simulink model "FOSTWIN"  (R2022a)
settings: Solver=FixedStepAuto  StartTime=0.0  StopTime=30  FixedStep=Ts  RelTol=1e-3
values from neighbouring files (symbols this model uses):
  D = (1+2*k*h/(sinh(2*k*h)))*tanh(k*h)    [SIDWaveGenerator.m]
  initTime = 2    [initModels_GUI.m]
  Kt = 0.943    [initModels_GUI.m]
  lpFreqCurrent = 50    [initModels_GUI.m]
  lpFreqVelocity = 50    [initModels_GUI.m]
  maxCurrent = 15    [initModels_GUI.m]
  maxFaultCount = 3    [initModels_GUI.m]
  param1 = 5    [initModels_GUI.m]    (also in starttarget.m = param1New)
  param2 = 5    [initModels_GUI.m]    (also in starttarget.m = param2New)
  param3 = 10    [initModels_GUI.m]    (also in starttarget.m = param3New)
  param4 = 10    [initModels_GUI.m]    (also in starttarget.m = param4New)
  safeDamping = 2.5    [initModels_GUI.m]
  safeTime = 20    [initModels_GUI.m]
  stableTime = 3    [initModels_GUI.m]
  Ts = 1/1000    (= 0.001)    [FOSTWINctrlPost.m]    (also in initModels_GUI.m)
  waveH = 1    [SIDWaveGenerator.m]    (also in initModels_GUI.m = 0.136; starttarget.m = waveHNew)
undefined symbols (not defined in the file or in its folder): control_id_twin4, ctrl2TwinStruct, ctrlParam1, ctrlParam2, ctrlParam3, ctrlParam4, ctrlParamStruct, curAft, curBow, dataID_twin6, param5, paramStruct, pcktID, posFlapAft, posFlapBow, SimStateMsg, state, twin2CtrlStruct
libraries: simulink x48, slrealtimeutilitieslib x24, slrealtimeethercatlib x6, slrealtimeloglib x4, dspstat3 x3, slrealtimeiplib x3, slrealtimetgmanagement x1
(part 1 of 2)
settings Model: Creator=HWRL user  LastModifiedBy=jspin
settings SolverCC: ConcurrentTasks=on  PositivePriorityOrder=on
settings DataIOCC: ExternalInput=FexAft, FexBow  TimeSaveName=toutTop  OutputSaveName=youtTop
settings OptimizationCC: BlockReduction=off  OptimizeBlockIOStorage=off  ZeroExternalMemoryAtStartup=off  ZeroInternalMemoryAtStartup=off
settings DebuggingCC: TasksWithSamePriorityMsg=none  UnconnectedInputMsg=warning  UnconnectedOutputMsg=warning  UnconnectedLineMsg=warning
settings HardwareCC: ProdBitPerLong=64  ProdLongLongMode=on  ProdHWDeviceType=Intel->x86-64 (Linux 64)
settings RTWCC: Description=Generic Real-Time Target  RTWVerbose=off  Toolchain=Simulink Real-Time Toolchain  BuildConfiguration=Faster Runs  TargetLang=C++  DLArmComputeVersion=19.05
settings GRTTargetCC: TargetLangStandard=C++03 (ISO)  CodeInterfacePackaging=C++ class

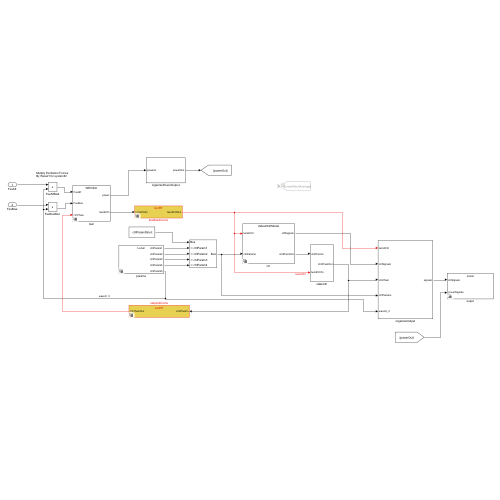
[thumbnail: Simulink's stored preview of the top-level diagram]
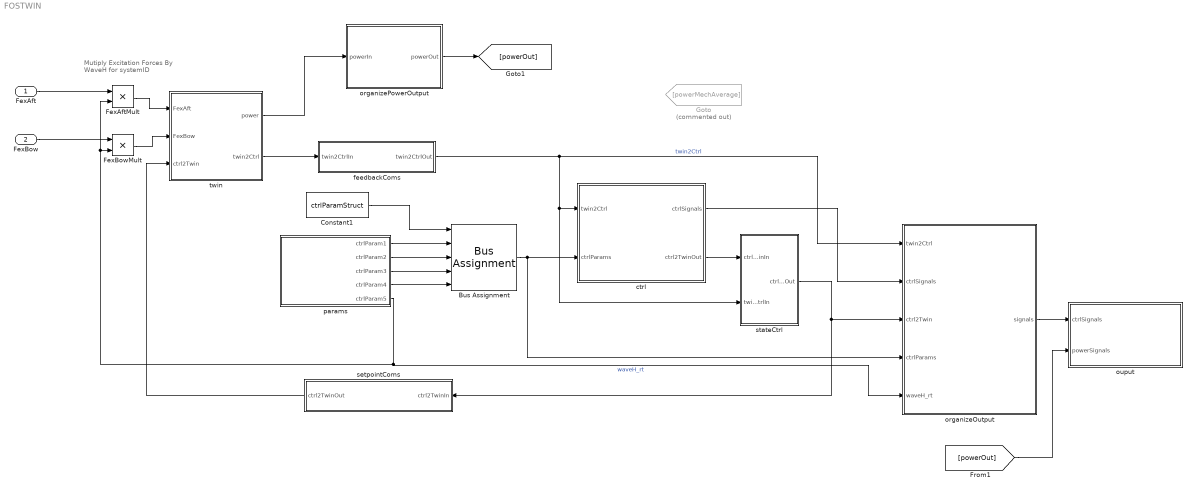
== system FOSTWIN ==
  note: Mutiply Excitation Forces
      | By WaveH for systemID
  FexAft : Inport  Interpolate=off
  FexBow : Inport  Port=2  Interpolate=off
  Bus Assignment : BusAssignment  AssignedSignals=ctrlParam1,ctrlParam2,ctrlParam3,ctrlParam4
  Constant1 : Constant  Value=ctrlParamStruct  VectorParams1D=off  OutDataTypeStr=Bus: ctrlParamBus
  FexAftMult : Product
  FexBowMult : Product
  Goto : Goto  Commented=on  GotoTag=powerMechAverage
  ctrl : Subsystem  Variant=on  VariantControlMode=label  LabelModeActiveChoice=defaultCtrlModel
  feedbackComs : Subsystem  Variant=on  VariantControlMode=label  LabelModeActiveChoice=nonRT
  organizeOutput : Subsystem
  organizePowerOutput : Subsystem
  ouput : Subsystem  Variant=on  VariantControlMode=label  LabelModeActiveChoice=Local
  params : Subsystem  Variant=on  VariantControlMode=label  LabelModeActiveChoice=Local
  setpointComs : Subsystem  Variant=on  VariantControlMode=label  LabelModeActiveChoice=nonRT
  stateCtrl : Subsystem
  twin : Subsystem  Variant=on  VariantControlMode=label  LabelModeActiveChoice=WECSim
  wires:
  FexBowMult/1 -> twin/2(FexBow)
  params/5(ctrlParam5) -> organizeOutput/5(waveH_rt), FexAftMult/2, FexBowMult/2  "waveH_rt"
  FexAftMult/1 -> twin/1(FexAft)
  setpointComs/1(ctrl2TwinOut) -> twin/3(ctrl2Twin)
  twin/2(twin2Ctrl) -> feedbackComs/1(twin2CtrlIn)
  feedbackComs/1(twin2CtrlOut) -> organizeOutput/1(twin2Ctrl), ctrl/1(twin2Ctrl), stateCtrl/2(twin2CtrlIn)  "twin2Ctrl"
  stateCtrl/1(ctrl2TwinOut) -> setpointComs/1(ctrl2TwinIn), organizeOutput/3(ctrl2Twin)
  Constant1/1 -> Bus Assignment/1
  Bus Assignment/1 -> organizeOutput/4(ctrlParams), ctrl/2(ctrlParams)
  organizeOutput/1(signals) -> ouput/1(ctrlSignals)
  twin/1(power) -> organizePowerOutput/1(powerIn)
  organizePowerOutput/1(powerOut) -> [powerOut]
  params/1(ctrlParam1) -> Bus Assignment/2
  params/2(ctrlParam2) -> Bus Assignment/3
  params/4(ctrlParam4) -> Bus Assignment/5
  [powerOut] -> ouput/2(powerSignals)
  ctrl/1(ctrlSignals) -> organizeOutput/2(ctrlSignals)
  ctrl/2(ctrl2TwinOut) -> stateCtrl/1(ctrl2TwinIn)
  params/3(ctrlParam3) -> Bus Assignment/4
  FexAft/1 -> FexAftMult/1
  FexBow/1 -> FexBowMult/1

== system FOSTWIN/ctrl ==
  note: 1) Add Subsystem or Model blocks as valid variant choices.
      | 2) You cannot connect blocks at this level. At simulation, connectivity is automatically
      | determined, based on the active variant and port name matching.
  twin2Ctrl : Inport  OutDataTypeStr=Bus: twin2CtrlBus
  ctrlParams : Inport  Port=2  OutDataTypeStr=Bus: ctrlParamBus
  defaultCtrlModel : ModelReference  ModelNameDialog=defaultCtrlModel  SimulationMode=Normal  VariantControl=defaultCtrlModel  OverrideUsingVariant=defaultCtrlModel  ModelReferenceVersion=4.551
  userCtrlModel : ModelReference  ModelNameDialog=ctrlStarter  SimulationMode=Normal  VariantControl=userCtrlModel  ModelReferenceVersion=3.17
  ctrlSignals : Outport  OutDataTypeStr=Bus: ctrlSignalBus
  ctrl2TwinOut : Outport  Port=2  OutDataTypeStr=Bus: ctrl2TwinBus

== system FOSTWIN/feedbackComs ==
  note: 1) Add Subsystem or Model blocks as valid variant choices.
      | 2) You cannot connect blocks at this level. At simulation, connectivity is automatically
      | determined, based on the active variant and port name matching.
  twin2CtrlIn : Inport  OutDataTypeStr=Bus: twin2CtrlBus
  nonRT : Subsystem  VariantControl=nonRT
  singleSpeedgoat : Subsystem  VariantControl=singleSpeedgoat
  twoSpeedgoats : Subsystem  VariantControl=twoSpeedgoats
  twin2CtrlOut : Outport  OutDataTypeStr=Bus: twin2CtrlBus

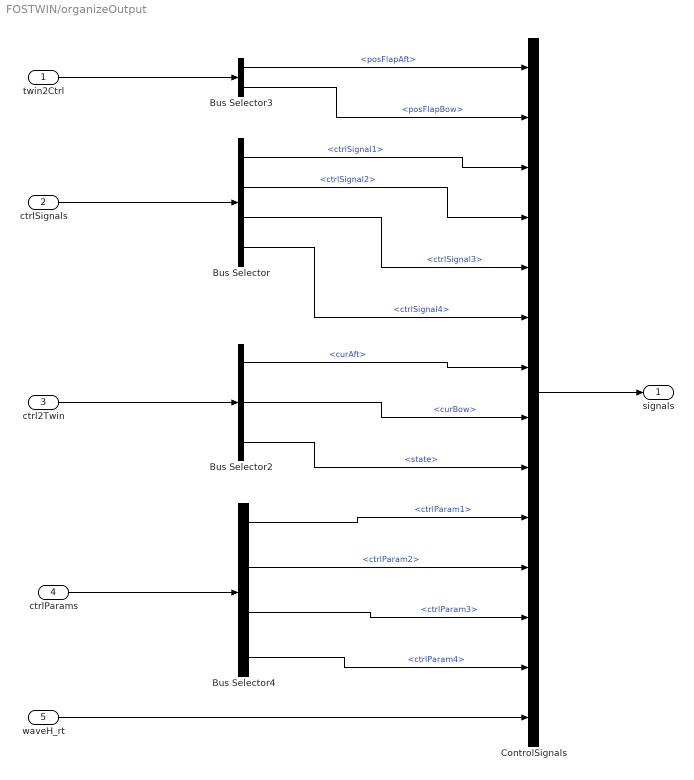
== system FOSTWIN/organizeOutput ==
  twin2Ctrl : Inport  OutDataTypeStr=Bus: twin2CtrlBus
  ctrlSignals : Inport  Port=2  OutDataTypeStr=Bus: ctrlSignalBus
  ctrl2Twin : Inport  Port=3
  ctrlParams : Inport  Port=4
  waveH_rt : Inport  Port=5
  Bus Selector : BusSelector  OutputSignals=ctrlSignal1,ctrlSignal2,ctrlSignal3,ctrlSignal4
  Bus Selector2 : BusSelector  OutputSignals=curAft,curBow,state
  Bus Selector3 : BusSelector  OutputSignals=posFlapAft,posFlapBow
  Bus Selector4 : BusSelector  OutputSignals=ctrlParam1,ctrlParam2,ctrlParam3,ctrlParam4
  ControlSignals : BusCreator  Inputs=14
  signals : Outport
  wires:
  Bus Selector2/2 -> ControlSignals/8  "<curBow>"
  waveH_rt/1 -> ControlSignals/14
  Bus Selector4/1 -> ControlSignals/10  "<ctrlParam1>"
  Bus Selector2/1 -> ControlSignals/7  "<curAft>"
  ctrlParams/1 -> Bus Selector4/1
  ControlSignals/1 -> signals/1
  ctrl2Twin/1 -> Bus Selector2/1
  twin2Ctrl/1 -> Bus Selector3/1
  Bus Selector3/1 -> ControlSignals/1  "<posFlapAft>"
  Bus Selector3/2 -> ControlSignals/2  "<posFlapBow>"
  ctrlSignals/1 -> Bus Selector/1
  Bus Selector/1 -> ControlSignals/3  "<ctrlSignal1>"
  Bus Selector/2 -> ControlSignals/4  "<ctrlSignal2>"
  Bus Selector/3 -> ControlSignals/5  "<ctrlSignal3>"
  Bus Selector/4 -> ControlSignals/6  "<ctrlSignal4>"
  Bus Selector4/2 -> ControlSignals/11  "<ctrlParam2>"
  Bus Selector4/3 -> ControlSignals/12  "<ctrlParam3>"
  Bus Selector4/4 -> ControlSignals/13  "<ctrlParam4>"
  Bus Selector2/3 -> ControlSignals/9  "<state>"

== system FOSTWIN/organizePowerOutput ==
  powerIn : Inport  OutDataTypeStr=Bus: powerBus
  Bus Creator : BusCreator  Inputs=8
  Bus Selector : BusSelector  OutputSignals=powerMechAft,powerMechBow,powerMechTotal,powerI2R,powerNet
  Bus Selector1 : BusSelector  OutputSignals=powerMechTotal
  Bus Selector2 : BusSelector  OutputSignals=powerNet
  Mean : dspstat3/Mean  run=on  InputProcessing=Columns as channels (frame based)  reset_popup=None  directionMode=Each column  dimension=1  roiEnable=off  roiType=Rectangles  roiPortion=Entire ROI  roiOutput=Individual statistics for each ROI  roiFlag=off  roundingMode=Floor  overflowMode=off  outputDataTypeStr=Inherit: Same as accumulator  outputMin=[]  outputMax=[]  outputLastDataTypeStr=Inherit: Same as accumulator
  Moving Average : dspstat3/Moving Average  Method=Sliding window  ForgettingFactorPort=off  SpecifyWindowLength=on  WindowLength=numSteps  ForgettingFactor=0.9  SimulateUsing=Code generation
  Moving Average1 : dspstat3/Moving Average  Method=Sliding window  ForgettingFactorPort=off  SpecifyWindowLength=on  WindowLength=numSteps  ForgettingFactor=0.9  SimulateUsing=Code generation
  powerOut : Outport
  wires:
  Bus Creator/1 -> powerOut/1
  Bus Selector/1 -> Bus Creator/1  "<powerMechAft>"
  Bus Selector1/1 -> Moving Average/1  "<powerMechTotal>"
  Bus Selector/3 -> Bus Creator/3  "<powerMechTotal>"
  Bus Selector/2 -> Bus Creator/2  "<powerMechBow>"
  Bus Selector/4 -> Bus Creator/4  "<powerI2R>"
  Bus Selector/5 -> Bus Creator/5  "<powerNet>"
  Moving Average/1 -> Bus Creator/6  "powerMechAverage"
  Bus Selector2/1 -> Moving Average1/1, Mean/1  "<powerNet>"
  Mean/1 -> Bus Creator/7  "powerNetMean"
  powerIn/1 -> Bus Selector2/1, Bus Selector1/1, Bus Selector/1
  Moving Average1/1 -> Bus Creator/8  "powerNetMovingAverage"

== system FOSTWIN/ouput ==
  note: 1) Add Subsystem or Model blocks as valid variant choices.
      | 2) You cannot connect blocks at this level. At simulation, connectivity is automatically
      | determined, based on the active variant and port name matching.
  ctrlSignals : Inport
  powerSignals : Inport  Port=2
  Local : Subsystem  VariantControl=Local
  Remote : Subsystem  VariantControl=Remote

== system FOSTWIN/params ==
  note: 1) Add Subsystem or Model blocks as valid variant choices.
      | 2) You cannot connect blocks at this level. At simulation, connectivity is automatically
      | determined, based on the active variant and port name matching.
  Local : Subsystem  VariantControl=Local
  Remote : Subsystem  VariantControl=Remote
  ctrlParam1 : Outport
  ctrlParam2 : Outport  Port=2
  ctrlParam3 : Outport  Port=3
  ctrlParam4 : Outport  Port=4
  ctrlParam5 : Outport  Port=5

== system FOSTWIN/setpointComs ==
  note: 1) Add Subsystem or Model blocks as valid variant choices.
      | 2) You cannot connect blocks at this level. At simulation, connectivity is automatically
      | determined, based on the active variant and port name matching.
  ctrl2TwinIn : Inport  OutDataTypeStr=Bus: ctrl2TwinBus
  nonRT : Subsystem  VariantControl=nonRT
  singleSpeedgoat : Subsystem  VariantControl=singleSpeedgoat
  twoSpeedgoats : Subsystem  VariantControl=twoSpeedgoats
  ctrl2TwinOut : Outport  OutDataTypeStr=Bus: ctrl2TwinBus

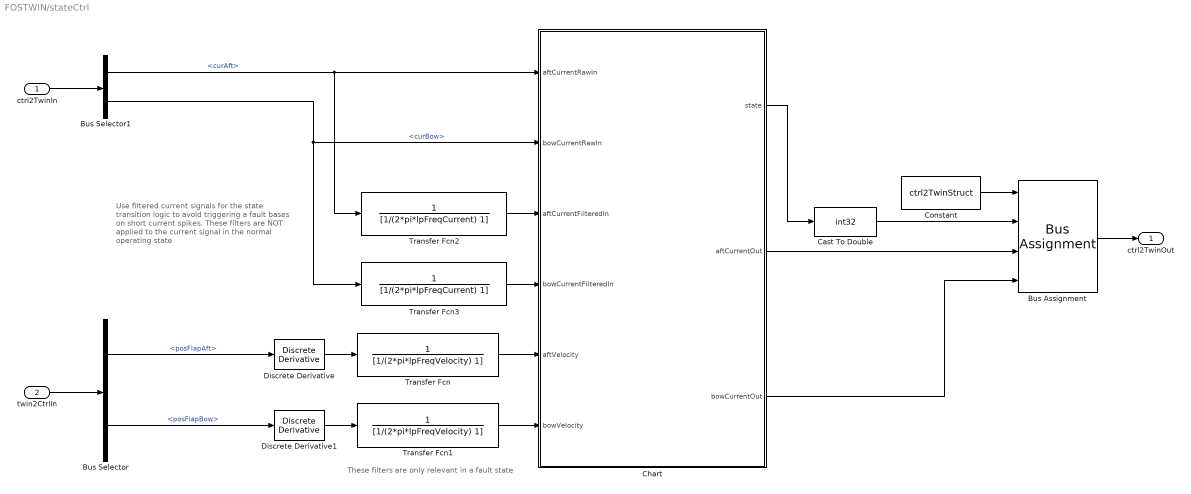
== system FOSTWIN/stateCtrl ==
  note: These filters are only relevant in a fault state
  note: Use filtered current signals for the state transition logic to avoid triggering a fault bases on short current spikes. These filters are NOT applied to the current signal in the normal operating state
  ctrl2TwinIn : Inport  OutDataTypeStr=Bus: ctrl2TwinBus
  twin2CtrlIn : Inport  Port=2  OutDataTypeStr=Bus: twin2CtrlBus
  Bus Assignment : BusAssignment  AssignedSignals=state,curAft,curBow
  Bus Selector : BusSelector  OutputSignals=posFlapAft,posFlapBow
  Bus Selector1 : BusSelector  OutputSignals=curAft,curBow
  Cast To Double : DataTypeConversion  OutDataTypeStr=int32  SaturateOnIntegerOverflow=off  RndMeth=Floor
  Chart : Stateflow chart  TreatAsAtomicUnit=on
  Constant : Constant  Value=ctrl2TwinStruct  OutDataTypeStr=Bus: ctrl2TwinBus
  Discrete Derivative : simulink/Discrete/Discrete Derivative  gainval=1.0  ICPrevScaledInput=0.0  OutMin=[]  OutMax=[]  OutDataType=fixdt(1, 16)  OutScaling=2^-10  DoSatur=off
  Discrete Derivative1 : simulink/Discrete/Discrete Derivative  gainval=1.0  ICPrevScaledInput=0.0  OutMin=[]  OutMax=[]  OutDataType=fixdt(1, 16)  OutScaling=2^-10  DoSatur=off
  Transfer Fcn : TransferFcn  Denominator=[1/(2*pi*lpFreqVelocity) 1]
  Transfer Fcn1 : TransferFcn  Denominator=[1/(2*pi*lpFreqVelocity) 1]
  Transfer Fcn2 : TransferFcn  Denominator=[1/(2*pi*lpFreqCurrent) 1]
  Transfer Fcn3 : TransferFcn  Denominator=[1/(2*pi*lpFreqCurrent) 1]
  ctrl2TwinOut : Outport  OutDataTypeStr=Bus: ctrl2TwinBus
  wires:
  Chart/1(state) -> Cast To Double/1
  Discrete Derivative/1 -> Transfer Fcn/1
  Discrete Derivative1/1 -> Transfer Fcn1/1
  Chart/3(bowCurrentOut) -> Bus Assignment/4
  Transfer Fcn/1 -> Chart/5(aftVelocity)
  Bus Selector1/1 -> Transfer Fcn2/1, Chart/1(aftCurrentRawIn)  "<curAft>"
  Transfer Fcn2/1 -> Chart/3(aftCurrentFilteredIn)
  Transfer Fcn3/1 -> Chart/4(bowCurrentFilteredIn)
  Transfer Fcn1/1 -> Chart/6(bowVelocity)
  twin2CtrlIn/1 -> Bus Selector/1
  Bus Selector/1 -> Discrete Derivative/1  "<posFlapAft>"
  Bus Selector/2 -> Discrete Derivative1/1  "<posFlapBow>"
  ctrl2TwinIn/1 -> Bus Selector1/1
  Bus Selector1/2 -> Transfer Fcn3/1, Chart/2(bowCurrentRawIn)  "<curBow>"
  Constant/1 -> Bus Assignment/1
  Chart/2(aftCurrentOut) -> Bus Assignment/3
  Bus Assignment/1 -> ctrl2TwinOut/1
  Cast To Double/1 -> Bus Assignment/2

== system FOSTWIN/twin ==
  note: 1) Add Subsystem or Model blocks as valid variant choices.
      | 2) You cannot connect blocks at this level. At simulation, connectivity is automatically
      | determined, based on the active variant and port name matching.
  FexAft : Inport
  FexBow : Inport  Port=2
  ctrl2Twin : Inport  Port=3  OutDataTypeStr=Bus: ctrl2TwinBus
  WECSim : ModelReference  ModelNameDialog=FOSWEC_v2.slx  SimulationMode=Normal  VariantControl=WECSim  ModelReferenceVersion=5.147
  systemID : ModelReference  ModelNameDialog=systemID.slx  SimulationMode=Normal  VariantControl=systemID  ModelReferenceVersion=3.515
  power : Outport  OutDataTypeStr=Bus: powerBus
  twin2Ctrl : Outport  Port=2  OutDataTypeStr=Bus: twin2CtrlBus

== system FOSTWIN/feedbackComs/nonRT ==
  twin2CtrlIn : Inport  OutDataTypeStr=Bus: twin2CtrlBus
  Memory2 : Memory
  twin2CtrlOut : Outport  OutDataTypeStr=Bus: twin2CtrlBus
  wires:
  twin2CtrlIn/1 -> Memory2/1
  Memory2/1 -> twin2CtrlOut/1

== system FOSTWIN/feedbackComs/singleSpeedgoat ==
  twin2CtrlIn : Inport  OutDataTypeStr=Bus: twin2CtrlBus
  twin2CtrlOut : Outport  OutDataTypeStr=Bus: twin2CtrlBus
  wires:
  twin2CtrlIn/1 -> twin2CtrlOut/1

== system FOSTWIN/feedbackComs/twoSpeedgoats ==
  note: TODO: Change order (aft should generally be first)
  twin2CtrlIn : Inport  OutDataTypeStr=Bus: twin2CtrlBus
  Bus Assignment : BusAssignment  AssignedSignals=posFlapBow,posFlapAft
  Constant : Constant  Value=twin2CtrlStruct  OutDataTypeStr=Bus: twin2CtrlBus
  EtherCAT Init : slrealtimeethercatlib/EtherCAT Init  Priority=0  config_file=D:\src\SANDIA-OSU\FOSTWIN-Twin\esi\FOSTWIN_Secondary1.xml  device_id=0  pci_bus=0  pci_slot=0  pci_function=0  portnum=1  initstate=2  dctuning=2  enaDebug=2  enaDC=on  errLink=off  masterDbg=off  stateChgDbg=off  baseClock=off  masterCfg=off  logFile='c:\dbglog.txt'  sample_time=0.001000  DCMode=0
      settings: SourceProductBaseCode=XP
  EtherCAT PDO Receive : slrealtimeethercatlib/EtherCAT PDO Receive  Priority=2  sig_name=Box 1 (EL6695-0002).IO Inputs.P2S01  sig_offset=328  sig_type=double  type_size=64  sig_dim=1  device_id=0  sample_time=0.001000
      settings: SourceProductBaseCode=XP
  EtherCAT PDO Receive1 : slrealtimeethercatlib/EtherCAT PDO Receive  Priority=2  sig_name=Box 1 (EL6695-0002).IO Inputs.P2S02  sig_offset=392  sig_type=double  type_size=64  sig_dim=1  device_id=0  sample_time=0.001000
      settings: SourceProductBaseCode=XP
  Terminator : Terminator
  Terminator1 : Terminator
  twin2CtrlOut : Outport
  wires:
  EtherCAT Init/1 -> Terminator/1
  twin2CtrlIn/1 -> Terminator1/1
  Constant/1 -> Bus Assignment/1
  EtherCAT PDO Receive/1 -> Bus Assignment/2
  EtherCAT PDO Receive1/1 -> Bus Assignment/3
  Bus Assignment/1 -> twin2CtrlOut/1

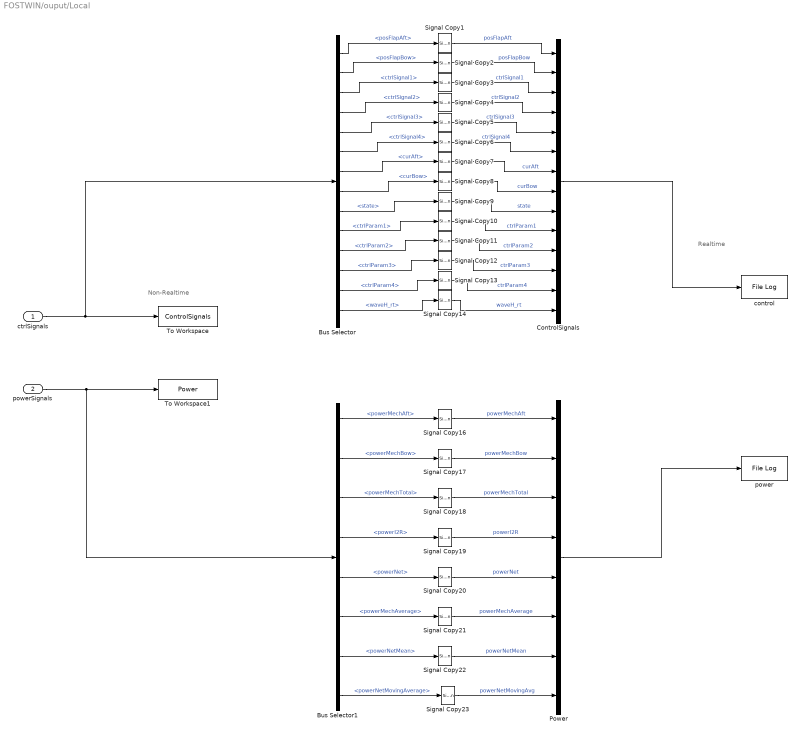
== system FOSTWIN/ouput/Local ==
  note: Non-Realtime
  note: Realtime
  ctrlSignals : Inport
  powerSignals : Inport  Port=2
  Bus Selector : BusSelector  OutputSignals=posFlapAft,posFlapBow,ctrlSignal1,ctrlSignal2,ctrlSignal3,ctrlSignal4,curAft,curBow,state,ctrlParam1,ctrlParam2,ctrlParam3,ctrlParam4,waveH_rt
  Bus Selector1 : BusSelector  OutputSignals=powerMechAft,powerMechBow,powerMechTotal,powerI2R,powerNet,powerMechAverage,powerNetMean,powerNetMovingAverage
  ControlSignals : BusCreator  Inputs=14
  Power : BusCreator  Inputs=8
  Signal Copy{1..14,16..23} (22 alike) : SignalConversion  OverrideOpt=off
  To Workspace : ToWorkspace  VariableName=ControlSignals  SaveFormat=Timeseries  SampleTime=-1
  To Workspace1 : ToWorkspace  VariableName=Power  SaveFormat=Timeseries  SampleTime=-1
  control : slrealtimeloglib/File Log  decimation=10  inputProcessing=Elements as channels (sample based)
      settings: SourceProductBaseCode=XP
  power : slrealtimeloglib/File Log  decimation=10  inputProcessing=Elements as channels (sample based)
      settings: SourceProductBaseCode=XP
  wires:
  ctrlSignals/1 -> Bus Selector/1, To Workspace/1
  powerSignals/1 -> Bus Selector1/1, To Workspace1/1
  Bus Selector/7 -> Signal Copy7/1  "<curAft>"
  Bus Selector/1 -> Signal Copy1/1  "<posFlapAft>"
  Bus Selector/2 -> Signal Copy2/1  "<posFlapBow>"
  Signal Copy1/1 -> ControlSignals/1  "posFlapAft"
  Signal Copy2/1 -> ControlSignals/2  "posFlapBow"
  Bus Selector/3 -> Signal Copy3/1  "<ctrlSignal1>"
  Bus Selector/4 -> Signal Copy4/1  "<ctrlSignal2>"
  Bus Selector/5 -> Signal Copy5/1  "<ctrlSignal3>"
  Bus Selector/6 -> Signal Copy6/1  "<ctrlSignal4>"
  Bus Selector/8 -> Signal Copy8/1  "<curBow>"
  Bus Selector/9 -> Signal Copy9/1  "<state>"
  Bus Selector/10 -> Signal Copy10/1  "<ctrlParam1>"
  Bus Selector/11 -> Signal Copy11/1  "<ctrlParam2>"
  Bus Selector/12 -> Signal Copy12/1  "<ctrlParam3>"
  Bus Selector/13 -> Signal Copy13/1  "<ctrlParam4>"
  Bus Selector/14 -> Signal Copy14/1  "<waveH_rt>"
  Signal Copy3/1 -> ControlSignals/3  "ctrlSignal1"
  Signal Copy4/1 -> ControlSignals/4  "ctrlSignal2"
  Signal Copy5/1 -> ControlSignals/5  "ctrlSignal3"
  Signal Copy6/1 -> ControlSignals/6  "ctrlSignal4"
  Signal Copy7/1 -> ControlSignals/7  "curAft"
  Signal Copy8/1 -> ControlSignals/8  "curBow"
  Signal Copy9/1 -> ControlSignals/9  "state"
  Signal Copy10/1 -> ControlSignals/10  "ctrlParam1"
  Signal Copy11/1 -> ControlSignals/11  "ctrlParam2"
  Signal Copy12/1 -> ControlSignals/12  "ctrlParam3"
  Signal Copy13/1 -> ControlSignals/13  "ctrlParam4"
  Signal Copy14/1 -> ControlSignals/14  "waveH_rt"
  ControlSignals/1 -> control/1
  Bus Selector1/6 -> Signal Copy21/1  "<powerMechAverage>"
  Bus Selector1/1 -> Signal Copy16/1  "<powerMechAft>"
  Bus Selector1/2 -> Signal Copy17/1  "<powerMechBow>"
  Bus Selector1/3 -> Signal Copy18/1  "<powerMechTotal>"
  Bus Selector1/4 -> Signal Copy19/1  "<powerI2R>"
  Bus Selector1/5 -> Signal Copy20/1  "<powerNet>"
  Signal Copy17/1 -> Power/2  "powerMechBow"
  Signal Copy18/1 -> Power/3  "powerMechTotal"
  Signal Copy19/1 -> Power/4  "powerI2R"
  Signal Copy20/1 -> Power/5  "powerNet"
  Signal Copy21/1 -> Power/6  "powerMechAverage"
  Power/1 -> power/1
  Signal Copy16/1 -> Power/1  "powerMechAft"
  Bus Selector1/7 -> Signal Copy22/1  "<powerNetMean>"
  Signal Copy22/1 -> Power/7  "powerNetMean"
  Bus Selector1/8 -> Signal Copy23/1  "<powerNetMovingAverage>"
  Signal Copy23/1 -> Power/8  "powerNetMovingAvg"

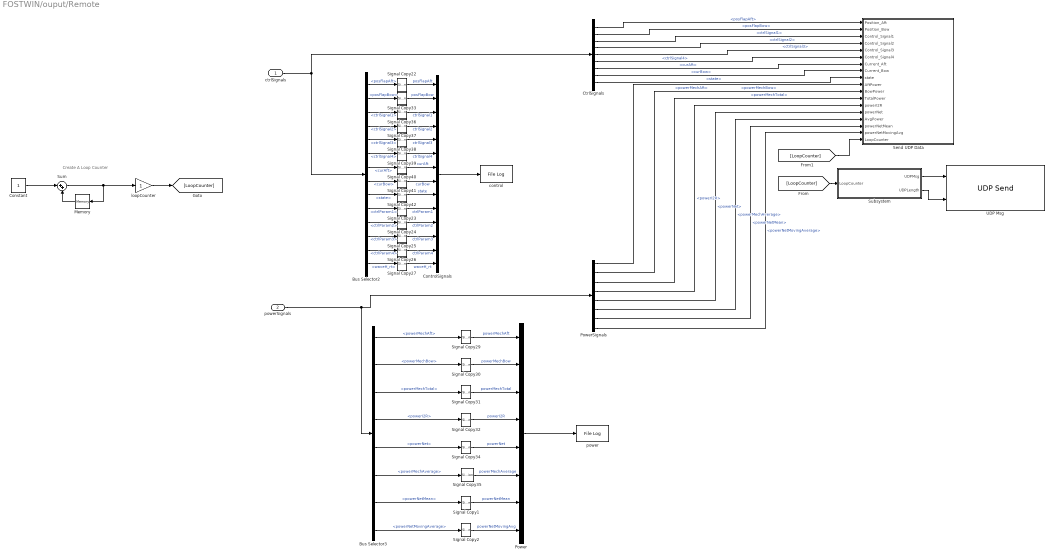
== system FOSTWIN/ouput/Remote ==
  note: Create A Loop Counter
  ctrlSignals : Inport
  powerSignals : Inport  Port=2
  Bus Selector2 : BusSelector  OutputSignals=posFlapAft,posFlapBow,ctrlSignal1,ctrlSignal2,ctrlSignal3,ctrlSignal4,curAft,curBow,state,ctrlParam1,ctrlParam2,ctrlParam3,ctrlParam4,waveH_rt
  Bus Selector3 : BusSelector  OutputSignals=powerMechAft,powerMechBow,powerMechTotal,powerI2R,powerNet,powerMechAverage,powerNetMean,powerNetMovingAverage
  Constant : Constant  SampleTime=Ts
  ControlSignals : BusCreator  Inputs=14
  CtrlSignals : BusSelector  OutputSignals=posFlapAft,posFlapBow,ctrlSignal1,ctrlSignal2,ctrlSignal3,ctrlSignal4,curAft,curBow,state
  Memory : Memory
  Power : BusCreator  Inputs=8
  PowerSignals : BusSelector  OutputSignals=powerMechAft,powerMechBow,powerMechTotal,powerI2R,powerNet,powerMechAverage,powerNetMean,powerNetMovingAverage
  Send UDP Data : Subsystem
  Signal Copy{1..2,22..27,29..42} (22 alike) : SignalConversion  OverrideOpt=off
  Subsystem : Subsystem
  Sum : Sum  Inputs=|++  OutDataTypeStr=uint32
  UDP Msg : slrealtimeiplib/UDP Send  useHostTargetConn=on  toAddress=iotIPaddr  toPort=iotRemoteMsgPort  sampleTime=Ts  enableMessage=off  ipAddress=10.10.10.15  localPort=iotLocalMsgPort
      settings: SourceProductBaseCode=XP
  control : slrealtimeloglib/File Log  decimation=10  inputProcessing=Elements as channels (sample based)
      settings: SourceProductBaseCode=XP
  loopCounter : Gain  ParamDataTypeStr=uint32  OutDataTypeStr=uint32
  power : slrealtimeloglib/File Log  decimation=10  inputProcessing=Elements as channels (sample based)
      settings: SourceProductBaseCode=XP
  wires:
  Subsystem/2(UDPLength) -> UDP Msg/2
  Sum/1 -> Memory/1, loopCounter/1
  Memory/1 -> Sum/2
  Constant/1 -> Sum/1
  Subsystem/1(UDPMsg) -> UDP Msg/1
  ctrlSignals/1 -> Bus Selector2/1, CtrlSignals/1
  CtrlSignals/1 -> Send UDP Data/1(Position_Aft)  "<posFlapAft>"
  loopCounter/1 -> [LoopCounter]
  [LoopCounter] -> Subsystem/1(LoopCounter)
  [LoopCounter] -> Send UDP Data/18(LoopCounter)
  CtrlSignals/2 -> Send UDP Data/2(Position_Bow)  "<posFlapBow>"
  CtrlSignals/3 -> Send UDP Data/3(Control_Signal1)  "<ctrlSignal1>"
  CtrlSignals/4 -> Send UDP Data/4(Control_Signal2)  "<ctrlSignal2>"
  CtrlSignals/5 -> Send UDP Data/5(Control_Signal3)  "<ctrlSignal3>"
  CtrlSignals/6 -> Send UDP Data/6(Control_Signal4)  "<ctrlSignal4>"
  CtrlSignals/7 -> Send UDP Data/7(Current_Aft)  "<curAft>"
  CtrlSignals/8 -> Send UDP Data/8(Current_Bow)  "<curBow>"
  CtrlSignals/9 -> Send UDP Data/9(state)  "<state>"
  powerSignals/1 -> PowerSignals/1, Bus Selector3/1
  PowerSignals/6 -> Send UDP Data/15(AvgPower)  "<powerMechAverage>"
  PowerSignals/5 -> Send UDP Data/14(powerNet)  "<powerNet>"
  PowerSignals/4 -> Send UDP Data/13(powerI2R)  "<powerI2R>"
  PowerSignals/3 -> Send UDP Data/12(TotalPower)  "<powerMechTotal>"
  PowerSignals/2 -> Send UDP Data/11(BowPower)  "<powerMechBow>"
  PowerSignals/1 -> Send UDP Data/10(AftPower)  "<powerMechAft>"
  Signal Copy42/1 -> ControlSignals/9  "state"
  Signal Copy31/1 -> Power/3  "powerMechTotal"
  Signal Copy32/1 -> Power/4  "powerI2R"
  Signal Copy30/1 -> Power/2  "powerMechBow"
  Signal Copy25/1 -> ControlSignals/12  "ctrlParam3"
  Signal Copy39/1 -> ControlSignals/6  "ctrlSignal4"
  Bus Selector3/5 -> Signal Copy34/1  "<powerNet>"
  Bus Selector2/5 -> Signal Copy38/1  "<ctrlSignal3>"
  Bus Selector3/2 -> Signal Copy30/1  "<powerMechBow>"
  Bus Selector2/3 -> Signal Copy36/1  "<ctrlSignal1>"
  Signal Copy36/1 -> ControlSignals/3  "ctrlSignal1"
  Signal Copy26/1 -> ControlSignals/13  "ctrlParam4"
  Bus Selector2/11 -> Signal Copy24/1  "<ctrlParam2>"
  Bus Selector3/4 -> Signal Copy32/1  "<powerI2R>"
  Signal Copy22/1 -> ControlSignals/1  "posFlapAft"
  Bus Selector2/2 -> Signal Copy33/1  "<posFlapBow>"
  Signal Copy34/1 -> Power/5  "powerNet"
  Signal Copy23/1 -> ControlSignals/10  "ctrlParam1"
  Bus Selector2/14 -> Signal Copy27/1  "<waveH_rt>"
  Signal Copy24/1 -> ControlSignals/11  "ctrlParam2"
  Bus Selector2/7 -> Signal Copy40/1  "<curAft>"
  Signal Copy41/1 -> ControlSignals/8  "curBow"
  Bus Selector3/3 -> Signal Copy31/1  "<powerMechTotal>"
  Signal Copy38/1 -> ControlSignals/5  "ctrlSignal3"
  Signal Copy37/1 -> ControlSignals/4  "ctrlSignal2"
  Signal Copy27/1 -> ControlSignals/14  "waveH_rt"
  Signal Copy40/1 -> ControlSignals/7  "curAft"
  Bus Selector2/9 -> Signal Copy42/1  "<state>"
  Bus Selector2/12 -> Signal Copy25/1  "<ctrlParam3>"
  Signal Copy35/1 -> Power/6  "powerMechAverage"
  Bus Selector2/6 -> Signal Copy39/1  "<ctrlSignal4>"
  Signal Copy29/1 -> Power/1  "powerMechAft"
  Bus Selector2/1 -> Signal Copy22/1  "<posFlapAft>"
  Bus Selector2/8 -> Signal Copy41/1  "<curBow>"
  Bus Selector2/10 -> Signal Copy23/1  "<ctrlParam1>"
  Signal Copy33/1 -> ControlSignals/2  "posFlapBow"
  Bus Selector3/1 -> Signal Copy29/1  "<powerMechAft>"
  Bus Selector2/13 -> Signal Copy26/1  "<ctrlParam4>"
  Bus Selector2/4 -> Signal Copy37/1  "<ctrlSignal2>"
  Power/1 -> power/1
  ControlSignals/1 -> control/1
  Bus Selector3/7 -> Signal Copy1/1  "<powerNetMean>"
  Signal Copy1/1 -> Power/7  "powerNetMean"
  PowerSignals/7 -> Send UDP Data/16(powerNetMean)  "<powerNetMean>"
  Bus Selector3/6 -> Signal Copy35/1  "<powerMechAverage>"
  Bus Selector3/8 -> Signal Copy2/1  "<powerNetMovingAverage>"
  Signal Copy2/1 -> Power/8  "powerNetMovingAvg"
  PowerSignals/8 -> Send UDP Data/17(powerNetMovingAvg)  "<powerNetMovingAverage>"

== system FOSTWIN/params/Local ==
  note: These Params are set in starttarget.m
  ControlParams : Subsystem  Variant=on  VariantControlMode=label  LabelModeActiveChoice=NonRealTime
  ctrlParam1 : Outport
  ctrlParam2 : Outport  Port=2
  ctrlParam3 : Outport  Port=3
  ctrlParam4 : Outport  Port=4
  ctrlParam5 : Outport  Port=5
  wires:
  ControlParams/1(ctrlParam1) -> ctrlParam1/1
  ControlParams/2(ctrlParam2) -> ctrlParam2/1
  ControlParams/3(ctrlParam3) -> ctrlParam3/1
  ControlParams/4(ctrlParam4) -> ctrlParam4/1
  ControlParams/5(ctrlParam5) -> ctrlParam5/1

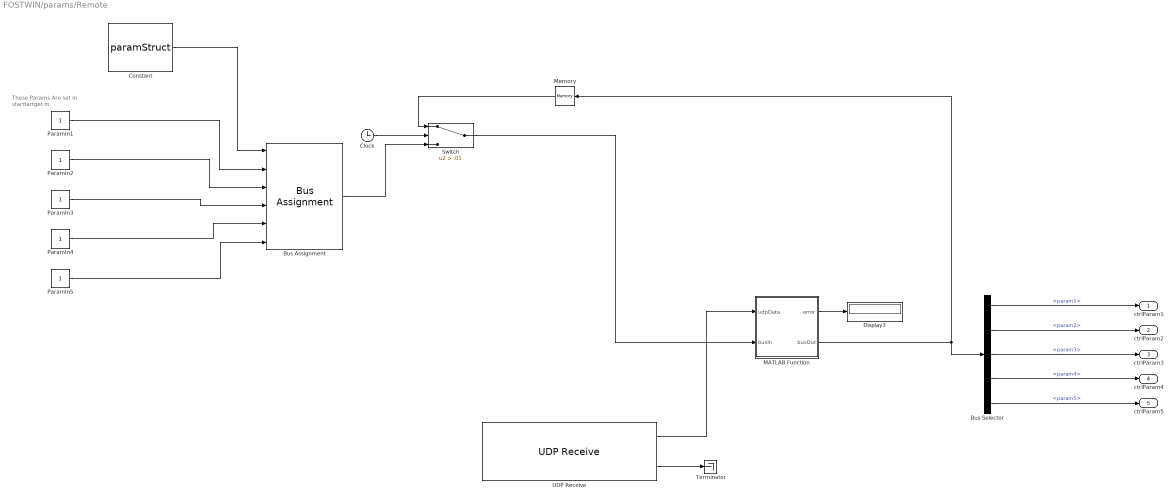
== system FOSTWIN/params/Remote ==
  note: These Params Are set in starttartget.m
  Bus Assignment : BusAssignment  AssignedSignals=param1,param2,param3,param4,param5
  Bus Selector : BusSelector  OutputSignals=param1,param2,param3,param4,param5
  Clock : Clock
  Constant : Constant  Value=paramStruct  VectorParams1D=off  OutDataTypeStr=Bus: slBus1
  Display3 : Display
  MATLAB Function : MATLAB Function  TreatAsAtomicUnit=on
  Memory : Memory
  ParamIn1 : Constant  SampleTime=Ts
  ParamIn2 : Constant  VectorParams1D=off  SampleTime=Ts
  ParamIn3 : Constant  SampleTime=Ts
  ParamIn4 : Constant  OutDataTypeStr=double  SampleTime=Ts
  ParamIn5 : Constant  OutDataTypeStr=double  SampleTime=Ts
  Switch : Switch  Criteria=u2 > Threshold  Threshold=.01  SaturateOnIntegerOverflow=off  InputSameDT=off
  Terminator : Terminator
  UDP Receive : slrealtimeiplib/UDP Receive  useHostTargetConn=on  ipAddress=10.10.10.15  localPort=iotLocalParamPort  rcvWidth=12  rcvFmAny=off  fmAddress=iotIPaddr  sampleTime=Ts  enableMessage=off  maxPackets=1
      settings: SourceProductBaseCode=XP
  ctrlParam1 : Outport
  ctrlParam2 : Outport  Port=2
  ctrlParam3 : Outport  Port=3
  ctrlParam4 : Outport  Port=4
  ctrlParam5 : Outport  Port=5
  wires:
  Bus Selector/4 -> ctrlParam4/1  "<param4>"
  Memory/1 -> Switch/1
  Bus Selector/1 -> ctrlParam1/1  "<param1>"
  UDP Receive/2 -> Terminator/1
  Bus Selector/5 -> ctrlParam5/1  "<param5>"
  UDP Receive/1 -> MATLAB Function/1(udpData)
  Clock/1 -> Switch/2
  ParamIn4/1 -> Bus Assignment/5
  MATLAB Function/1(error) -> Display3/1
  ParamIn2/1 -> Bus Assignment/3
  MATLAB Function/2(busOut) -> Memory/1, Bus Selector/1
  Switch/1 -> MATLAB Function/2(busIn)
  ParamIn3/1 -> Bus Assignment/4
  ParamIn1/1 -> Bus Assignment/2
  Bus Assignment/1 -> Switch/3
  ParamIn5/1 -> Bus Assignment/6
  Constant/1 -> Bus Assignment/1
  Bus Selector/3 -> ctrlParam3/1  "<param3>"
  Bus Selector/2 -> ctrlParam2/1  "<param2>"

== system FOSTWIN/setpointComs/nonRT ==
  ctrl2TwinIn : Inport  OutDataTypeStr=Bus: ctrl2TwinBus
  ctrl2TwinOut : Outport  OutDataTypeStr=Bus: ctrl2TwinBus
  wires:
  ctrl2TwinIn/1 -> ctrl2TwinOut/1

== system FOSTWIN/setpointComs/singleSpeedgoat ==
  ctrl2TwinIn : Inport  OutDataTypeStr=Bus: ctrl2TwinBus
  Delay2 : Delay  DelayLength=1
  ctrl2TwinOut : Outport  OutDataTypeStr=Bus: ctrl2TwinBus
  wires:
  ctrl2TwinIn/1 -> Delay2/1
  Delay2/1 -> ctrl2TwinOut/1

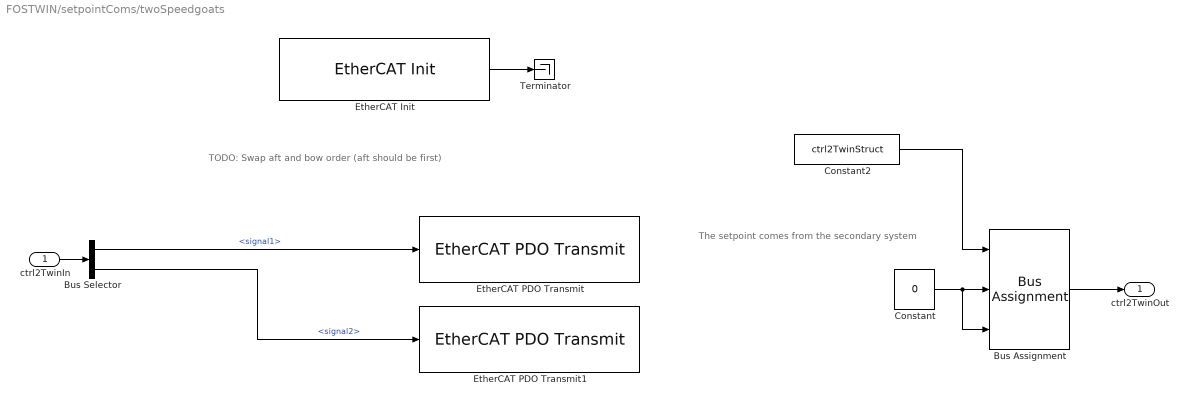
== system FOSTWIN/setpointComs/twoSpeedgoats ==
  note: TODO: Swap aft and bow order (aft should be first)
  note: The setpoint comes from the secondary system
  ctrl2TwinIn : Inport  OutDataTypeStr=Bus: ctrl2TwinBus
  Bus Assignment : BusAssignment  AssignedSignals=curAft,curBow
  Bus Selector : BusSelector  OutputSignals=signal1,signal2
  Constant : Constant  Value=0  VectorParams1D=off  SampleTime=-1
  Constant2 : Constant  Value=ctrl2TwinStruct  OutDataTypeStr=Bus: ctrl2TwinBus
  EtherCAT Init : slrealtimeethercatlib/EtherCAT Init  Priority=0  config_file=D:\src\SANDIA-OSU\FOSTWIN-Twin\esi\FOSTWIN-Primary1.xml  device_id=0  pci_bus=0  pci_slot=0  pci_function=0  portnum=1  initstate=2  dctuning=0  enaDebug=0  enaDC=on  errLink=off  masterDbg=off  stateChgDbg=off  baseClock=off  masterCfg=off  logFile='c:\dbglog.txt'  sample_time=0.001000  DCMode=0
      settings: SourceProductBaseCode=XP
  EtherCAT PDO Transmit : slrealtimeethercatlib/EtherCAT PDO Transmit  Priority=3  sig_name=Term 2 (EL6695).IO Outputs.P2S01  sig_offset=312  sig_type=double  type_size=64  sig_dim=1  device_id=0  sample_time=0.001000
      settings: SourceProductBaseCode=XP
  EtherCAT PDO Transmit1 : slrealtimeethercatlib/EtherCAT PDO Transmit  Priority=3  sig_name=Term 2 (EL6695).IO Outputs.P2S02  sig_offset=376  sig_type=double  type_size=64  sig_dim=1  device_id=0  sample_time=0.001000
      settings: SourceProductBaseCode=XP
  Terminator : Terminator
  ctrl2TwinOut : Outport
  wires:
  EtherCAT Init/1 -> Terminator/1
  Constant2/1 -> Bus Assignment/1
  Bus Assignment/1 -> ctrl2TwinOut/1
  Constant/1 -> Bus Assignment/3, Bus Assignment/2
  ctrl2TwinIn/1 -> Bus Selector/1
  Bus Selector/1 -> EtherCAT PDO Transmit/1  "<signal1>"
  Bus Selector/2 -> EtherCAT PDO Transmit1/1  "<signal2>"

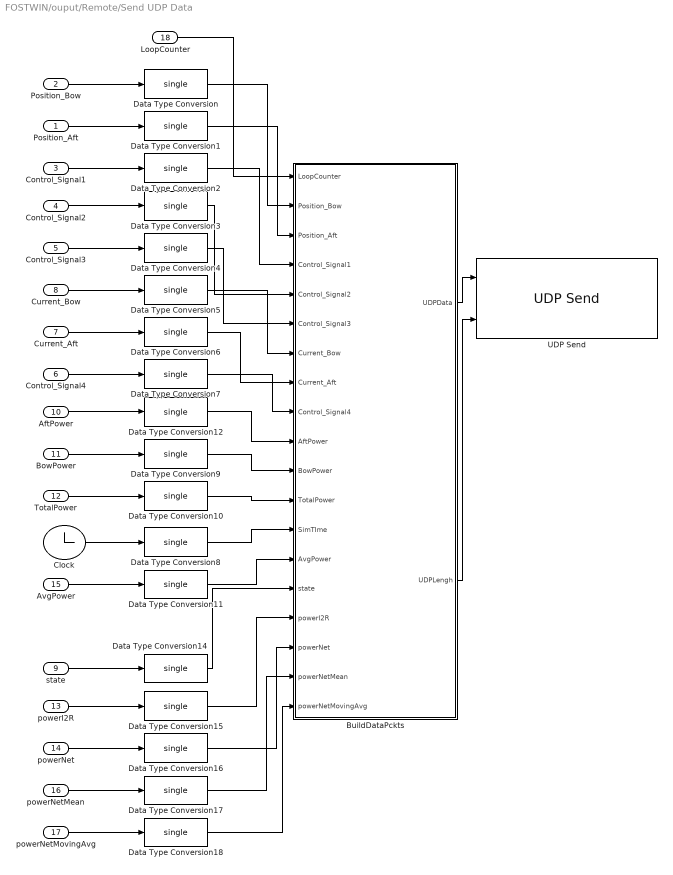
== system FOSTWIN/ouput/Remote/Send UDP Data ==
  Position_Aft : Inport
  Position_Bow : Inport  Port=2
  Control_Signal1 : Inport  Port=3
  Control_Signal2 : Inport  Port=4
  Control_Signal3 : Inport  Port=5
  Control_Signal4 : Inport  Port=6
  Current_Aft : Inport  Port=7
  Current_Bow : Inport  Port=8
  state : Inport  Port=9
  AftPower : Inport  Port=10
  BowPower : Inport  Port=11
  TotalPower : Inport  Port=12
  powerI2R : Inport  Port=13
  powerNet : Inport  Port=14
  AvgPower : Inport  Port=15
  powerNetMean : Inport  Port=16
  powerNetMovingAvg : Inport  Port=17
  LoopCounter : Inport  Port=18
  BuildDataPckts : Subsystem
  Clock : Clock
  Data Type Conversion{,1..12,14..18} (18 alike) : DataTypeConversion  OutDataTypeStr=single  SaturateOnIntegerOverflow=off  RndMeth=Floor
  UDP Send : slrealtimeiplib/UDP Send  useHostTargetConn=on  toAddress=iotIPaddr  toPort=iotRemoteDataPort  sampleTime=Ts  enableMessage=off  ipAddress=10.10.10.15  localPort=iotLocalDataPort
      settings: SourceProductBaseCode=XP
  wires:
  state/1 -> Data Type Conversion14/1
  Data Type Conversion1/1 -> BuildDataPckts/3(Position_Aft)
  Data Type Conversion16/1 -> BuildDataPckts/17(powerNet)
  Data Type Conversion15/1 -> BuildDataPckts/16(powerI2R)
  Data Type Conversion14/1 -> BuildDataPckts/15(state)
  powerI2R/1 -> Data Type Conversion15/1
  powerNet/1 -> Data Type Conversion16/1
  Data Type Conversion12/1 -> BuildDataPckts/10(AftPower)
  Data Type Conversion11/1 -> BuildDataPckts/14(AvgPower)
  Data Type Conversion10/1 -> BuildDataPckts/12(TotalPower)
  Data Type Conversion9/1 -> BuildDataPckts/11(BowPower)
  TotalPower/1 -> Data Type Conversion10/1
  AvgPower/1 -> Data Type Conversion11/1
  AftPower/1 -> Data Type Conversion12/1
  BowPower/1 -> Data Type Conversion9/1
  Data Type Conversion8/1 -> BuildDataPckts/13(SimTIme)
  Clock/1 -> Data Type Conversion8/1
  Data Type Conversion7/1 -> BuildDataPckts/9(Control_Signal4)
  Position_Aft/1 -> Data Type Conversion1/1
  LoopCounter/1 -> BuildDataPckts/1(LoopCounter)
  Current_Bow/1 -> Data Type Conversion5/1
  Control_Signal4/1 -> Data Type Conversion7/1
  Data Type Conversion5/1 -> BuildDataPckts/7(Current_Bow)
  Data Type Conversion6/1 -> BuildDataPckts/8(Current_Aft)
  Control_Signal3/1 -> Data Type Conversion4/1
  Current_Aft/1 -> Data Type Conversion6/1
  Data Type Conversion4/1 -> BuildDataPckts/6(Control_Signal3)
  Data Type Conversion3/1 -> BuildDataPckts/5(Control_Signal2)
  Control_Signal2/1 -> Data Type Conversion3/1
  Control_Signal1/1 -> Data Type Conversion2/1
  Data Type Conversion2/1 -> BuildDataPckts/4(Control_Signal1)
  Data Type Conversion/1 -> BuildDataPckts/2(Position_Bow)
  Position_Bow/1 -> Data Type Conversion/1
  BuildDataPckts/1(UDPData) -> UDP Send/1
  BuildDataPckts/2(UDPLengh) -> UDP Send/2
  powerNetMean/1 -> Data Type Conversion17/1
  Data Type Conversion17/1 -> BuildDataPckts/18(powerNetMean)
  powerNetMovingAvg/1 -> Data Type Conversion18/1
  Data Type Conversion18/1 -> BuildDataPckts/19(powerNetMovingAvg)

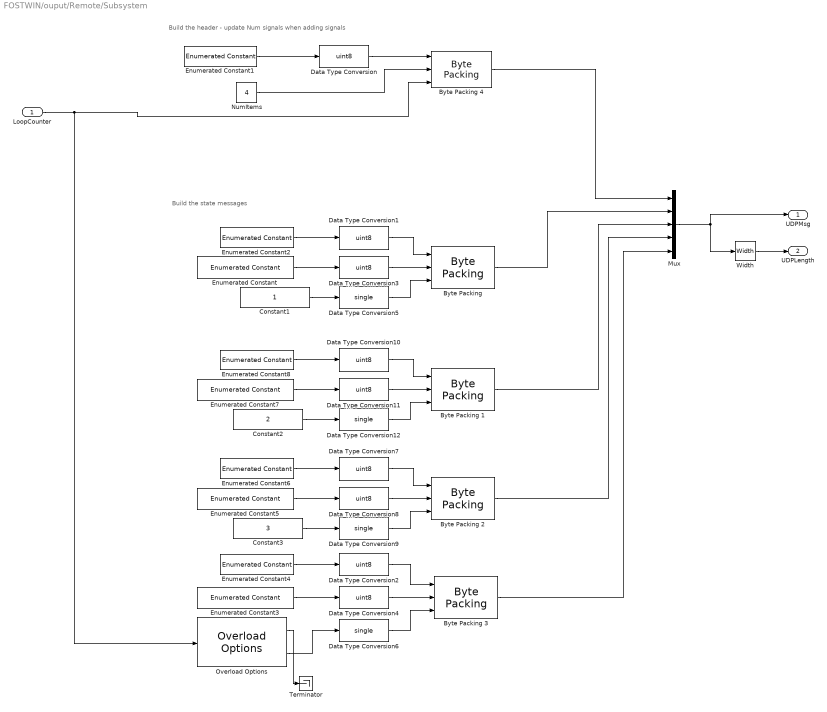
== system FOSTWIN/ouput/Remote/Subsystem ==
  note: Build the state messages
  note: Build the header - update Num signals when adding signals
  LoopCounter : Inport
  Byte Packing {,1..4} (5 alike) : slrealtimeutilitieslib/Byte Packing
  Constant1 : Constant
  Constant2 : Constant  Value=2
  Constant3 : Constant  Value=3
  Data Type Conversion{,1..4,7..8,10..11} (9 alike) : DataTypeConversion  OutDataTypeStr=uint8  SaturateOnIntegerOverflow=off  RndMeth=Floor
  Data Type Conversion{5..6,9,12} (4 alike) : DataTypeConversion  OutDataTypeStr=single  SaturateOnIntegerOverflow=off  RndMeth=Floor
  Enumerated Constant : simulink/Sources/Enumerated Constant  OutDataTypeStr=Enum: SimStateMsg  Value=SimStateMsg.eCATState  SampleTime=inf
  Enumerated Constant1 : simulink/Sources/Enumerated Constant  OutDataTypeStr=Enum: pcktID  Value=pcktID.header  SampleTime=inf
  Enumerated Constant{2,4,6,8} (4 alike) : simulink/Sources/Enumerated Constant  OutDataTypeStr=Enum: pcktID  Value=pcktID.stateMsg  SampleTime=inf
  Enumerated Constant3 : simulink/Sources/Enumerated Constant  OutDataTypeStr=Enum: SimStateMsg  Value=SimStateMsg.cpuTET  SampleTime=inf
  Enumerated Constant5 : simulink/Sources/Enumerated Constant  OutDataTypeStr=Enum: SimStateMsg  Value=SimStateMsg.eCATLastErr  SampleTime=inf
  Enumerated Constant7 : simulink/Sources/Enumerated Constant  OutDataTypeStr=Enum: SimStateMsg  Value=SimStateMsg.eCATErr  SampleTime=inf
  Mux : Mux  Inputs=5
  NumItems : Constant  Value=4  OutDataTypeStr=uint8
  Overload Options : slrealtimetgmanagement/Overload Options  startupDur=60  startupDurSrc=Tunable Parameter  maxOverload=200  maxOverloadSrc=Tunable Parameter  TETFlag=on
      settings: SourceProductBaseCode=XP
  Terminator : Terminator
  Width : Width
  UDPMsg : Outport
  UDPLength : Outport  Port=2
  wires:
  Constant2/1 -> Data Type Conversion12/1
  NumItems/1 -> Byte Packing 4/2
  Data Type Conversion9/1 -> Byte Packing 2/3
  Constant3/1 -> Data Type Conversion9/1
  Enumerated Constant2/1 -> Data Type Conversion1/1
  Constant1/1 -> Data Type Conversion5/1
  Enumerated Constant7/1 -> Data Type Conversion11/1
  Data Type Conversion2/1 -> Byte Packing 3/1
  Enumerated Constant4/1 -> Data Type Conversion2/1
  Data Type Conversion4/1 -> Byte Packing 3/2
  Enumerated Constant6/1 -> Data Type Conversion7/1
  Mux/1 -> UDPMsg/1, Width/1
  Byte Packing 1/1 -> Mux/3
  Width/1 -> UDPLength/1
  Data Type Conversion5/1 -> "Byte Packing "/3
  Data Type Conversion12/1 -> Byte Packing 1/3
  "Byte Packing "/1 -> Mux/2
  Data Type Conversion3/1 -> "Byte Packing "/2
  Data Type Conversion6/1 -> Byte Packing 3/3
  Data Type Conversion8/1 -> Byte Packing 2/2
  Enumerated Constant3/1 -> Data Type Conversion4/1
  Enumerated Constant8/1 -> Data Type Conversion10/1
  Data Type Conversion11/1 -> Byte Packing 1/2
  Enumerated Constant5/1 -> Data Type Conversion8/1
  Data Type Conversion1/1 -> "Byte Packing "/1
  Byte Packing 4/1 -> Mux/1
  Byte Packing 3/1 -> Mux/5
  Byte Packing 2/1 -> Mux/4
  Enumerated Constant/1 -> Data Type Conversion3/1
  Overload Options/2 -> Data Type Conversion6/1
  Data Type Conversion10/1 -> Byte Packing 1/1
  Data Type Conversion/1 -> Byte Packing 4/1
  Data Type Conversion7/1 -> Byte Packing 2/1
  Enumerated Constant1/1 -> Data Type Conversion/1
  Overload Options/1 -> Terminator/1
  LoopCounter/1 -> Overload Options/1, Byte Packing 4/3

== system FOSTWIN/params/Local/ControlParams ==
  note: 1) Add Subsystem or Model blocks as valid variant choices.
      | 2) You cannot connect blocks at this level. At simulation, connectivity is automatically
      | determined, based on the active variant and port name matching.
  NonRealTime : Subsystem  VariantControl=NonRealTime
  SingleSpeedgoat : Subsystem  VariantControl=SingleSpeedgoat
  ctrlParam1 : Outport
  ctrlParam2 : Outport  Port=2
  ctrlParam3 : Outport  Port=3
  ctrlParam4 : Outport  Port=4
  ctrlParam5 : Outport  Port=5

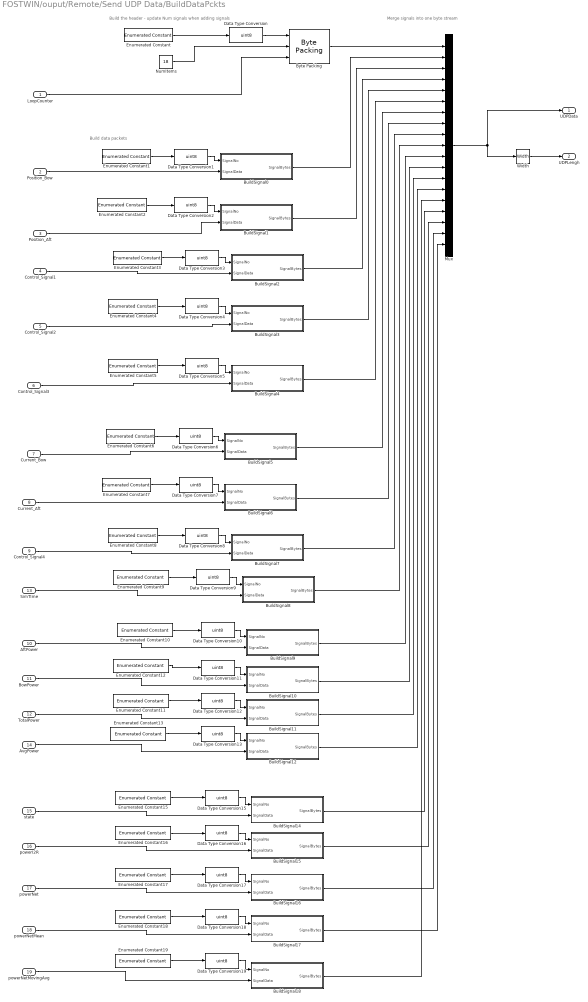
== system FOSTWIN/ouput/Remote/Send UDP Data/BuildDataPckts ==
  note: Merge signals into one byte stream
  note: Build data packets
  note: Build the header - update Num signals when adding signals
  LoopCounter : Inport
  Position_Bow : Inport  Port=2  OutDataTypeStr=single
  Position_Aft : Inport  Port=3  OutDataTypeStr=single
  Control_Signal1 : Inport  Port=4  OutDataTypeStr=single
  Control_Signal2 : Inport  Port=5  OutDataTypeStr=single
  Control_Signal3 : Inport  Port=6  OutDataTypeStr=single
  Current_Bow : Inport  Port=7  OutDataTypeStr=single
  Current_Aft : Inport  Port=8  OutDataTypeStr=single
  Control_Signal4 : Inport  Port=9  OutDataTypeStr=single
  AftPower : Inport  Port=10
  BowPower : Inport  Port=11
  TotalPower : Inport  Port=12
  SimTIme : Inport  Port=13
  AvgPower : Inport  Port=14
  state : Inport  Port=15
  powerI2R : Inport  Port=16
  powerNet : Inport  Port=17
  powerNetMean : Inport  Port=18
  powerNetMovingAvg : Inport  Port=19
  BuildSignal0 : Subsystem
  BuildSignal1 : Subsystem
  BuildSignal10 : Subsystem
  BuildSignal11 : Subsystem
  BuildSignal12 : Subsystem
  BuildSignal14 : Subsystem
  BuildSignal15 : Subsystem
  BuildSignal16 : Subsystem
  BuildSignal17 : Subsystem
  BuildSignal18 : Subsystem
  BuildSignal2 : Subsystem
  BuildSignal3 : Subsystem
  BuildSignal4 : Subsystem
  BuildSignal5 : Subsystem
  BuildSignal6 : Subsystem
  BuildSignal7 : Subsystem
  BuildSignal8 : Subsystem
  BuildSignal9 : Subsystem
  "Byte Packing " : slrealtimeutilitieslib/Byte Packing  MaskPackedDataType=uint8  MaskUnpackedDataTypes={'uint8','uint8','uint32'}  MaskAlignment=1
  Data Type Conversion{,1..13,15..19} (19 alike) : DataTypeConversion  OutDataTypeStr=uint8  SaturateOnIntegerOverflow=off  RndMeth=Floor
  Enumerated Constant : simulink/Sources/Enumerated Constant  OutDataTypeStr=Enum: pcktID  Value=pcktID.header  SampleTime=inf
  Enumerated Constant1 : simulink/Sources/Enumerated Constant  OutDataTypeStr=Enum: dataID_twin6  Value=dataID_twin6.position_bow  SampleTime=inf
  Enumerated Constant10 : simulink/Sources/Enumerated Constant  OutDataTypeStr=Enum: dataID_twin6  Value=dataID_twin6.power_aft  SampleTime=inf
  Enumerated Constant11 : simulink/Sources/Enumerated Constant  OutDataTypeStr=Enum: dataID_twin6  Value=dataID_twin6.power_total  SampleTime=inf
  Enumerated Constant12 : simulink/Sources/Enumerated Constant  OutDataTypeStr=Enum: dataID_twin6  Value=dataID_twin6.power_bow  SampleTime=inf
  Enumerated Constant13 : simulink/Sources/Enumerated Constant  OutDataTypeStr=Enum: dataID_twin6  Value=dataID_twin6.power_avg  SampleTime=inf
  Enumerated Constant15 : simulink/Sources/Enumerated Constant  OutDataTypeStr=Enum: dataID_twin6  Value=dataID_twin6.ctrl_state  SampleTime=inf
  Enumerated Constant16 : simulink/Sources/Enumerated Constant  OutDataTypeStr=Enum: dataID_twin6  Value=dataID_twin6.power_I2R  SampleTime=inf
  Enumerated Constant17 : simulink/Sources/Enumerated Constant  OutDataTypeStr=Enum: dataID_twin6  Value=dataID_twin6.power_net  SampleTime=inf
  Enumerated Constant18 : simulink/Sources/Enumerated Constant  OutDataTypeStr=Enum: dataID_twin6  Value=dataID_twin6.power_net_mean  SampleTime=inf
  Enumerated Constant19 : simulink/Sources/Enumerated Constant  OutDataTypeStr=Enum: dataID_twin6  Value=dataID_twin6.power_net_moving_avg  SampleTime=inf
  Enumerated Constant2 : simulink/Sources/Enumerated Constant  OutDataTypeStr=Enum: dataID_twin6  Value=dataID_twin6.position_aft  SampleTime=inf
  Enumerated Constant3 : simulink/Sources/Enumerated Constant  OutDataTypeStr=Enum: control_id_twin4  Value=control_id_twin4.signal1  SampleTime=inf
  Enumerated Constant4 : simulink/Sources/Enumerated Constant  OutDataTypeStr=Enum: control_id_twin4  Value=control_id_twin4.signal2  SampleTime=inf
  Enumerated Constant5 : simulink/Sources/Enumerated Constant  OutDataTypeStr=Enum: control_id_twin4  Value=control_id_twin4.signal3  SampleTime=inf
  Enumerated Constant6 : simulink/Sources/Enumerated Constant  OutDataTypeStr=Enum: dataID_twin6  Value=dataID_twin6.current_bow  SampleTime=inf
  Enumerated Constant7 : simulink/Sources/Enumerated Constant  OutDataTypeStr=Enum: dataID_twin6  Value=dataID_twin6.current_aft  SampleTime=inf
  Enumerated Constant8 : simulink/Sources/Enumerated Constant  OutDataTypeStr=Enum: control_id_twin4  Value=control_id_twin4.signal4  SampleTime=inf
  Enumerated Constant9 : simulink/Sources/Enumerated Constant  OutDataTypeStr=Enum: control_id_twin4  Value=control_id_twin4.SimTime  SampleTime=inf
  Mux : Mux  Inputs=19
  NumItems : Constant  Value=18  OutDataTypeStr=uint8
  Width : Width
  UDPData : Outport
  UDPLengh : Outport  Port=2
  wires:
  Width/1 -> UDPLengh/1
  Position_Bow/1 -> BuildSignal0/2(SignalData)
  "Byte Packing "/1 -> Mux/1
  BuildSignal0/1(SignalBytes) -> Mux/2
  BuildSignal1/1(SignalBytes) -> Mux/3
  Mux/1 -> UDPData/1, Width/1
  Data Type Conversion/1 -> "Byte Packing "/1
  Enumerated Constant/1 -> Data Type Conversion/1
  NumItems/1 -> "Byte Packing "/2
  LoopCounter/1 -> "Byte Packing "/3
  Position_Aft/1 -> BuildSignal1/2(SignalData)
  Data Type Conversion1/1 -> BuildSignal0/1(SignalNo)
  Data Type Conversion2/1 -> BuildSignal1/1(SignalNo)
  Enumerated Constant1/1 -> Data Type Conversion1/1
  Enumerated Constant2/1 -> Data Type Conversion2/1
  Control_Signal2/1 -> BuildSignal3/2(SignalData)
  BuildSignal2/1(SignalBytes) -> Mux/4
  Data Type Conversion4/1 -> BuildSignal3/1(SignalNo)
  Control_Signal3/1 -> BuildSignal4/2(SignalData)
  BuildSignal4/1(SignalBytes) -> Mux/6
  Data Type Conversion3/1 -> BuildSignal2/1(SignalNo)
  Data Type Conversion5/1 -> BuildSignal4/1(SignalNo)
  Enumerated Constant4/1 -> Data Type Conversion4/1
  Enumerated Constant5/1 -> Data Type Conversion5/1
  Control_Signal1/1 -> BuildSignal2/2(SignalData)
  Enumerated Constant3/1 -> Data Type Conversion3/1
  BuildSignal3/1(SignalBytes) -> Mux/5
  BuildSignal6/1(SignalBytes) -> Mux/8
  BuildSignal5/1(SignalBytes) -> Mux/7
  Enumerated Constant6/1 -> Data Type Conversion6/1
  Data Type Conversion7/1 -> BuildSignal6/1(SignalNo)
  Enumerated Constant7/1 -> Data Type Conversion7/1
  Current_Aft/1 -> BuildSignal6/2(SignalData)
  Data Type Conversion6/1 -> BuildSignal5/1(SignalNo)
  Current_Bow/1 -> BuildSignal5/2(SignalData)
  Enumerated Constant8/1 -> Data Type Conversion8/1
  Data Type Conversion8/1 -> BuildSignal7/1(SignalNo)
  Control_Signal4/1 -> BuildSignal7/2(SignalData)
  BuildSignal7/1(SignalBytes) -> Mux/9
  Data Type Conversion9/1 -> BuildSignal8/1(SignalNo)
  Enumerated Constant9/1 -> Data Type Conversion9/1
  SimTIme/1 -> BuildSignal8/2(SignalData)
  BuildSignal8/1(SignalBytes) -> Mux/10
  AftPower/1 -> BuildSignal9/2(SignalData)
  Enumerated Constant10/1 -> Data Type Conversion10/1
  Data Type Conversion10/1 -> BuildSignal9/1(SignalNo)
  Data Type Conversion11/1 -> BuildSignal10/1(SignalNo)
  Enumerated Constant12/1 -> Data Type Conversion11/1
  BowPower/1 -> BuildSignal10/2(SignalData)
  TotalPower/1 -> BuildSignal11/2(SignalData)
  Enumerated Constant11/1 -> Data Type Conversion12/1
  Data Type Conversion12/1 -> BuildSignal11/1(SignalNo)
  Data Type Conversion13/1 -> BuildSignal12/1(SignalNo)
  Enumerated Constant13/1 -> Data Type Conversion13/1
  AvgPower/1 -> BuildSignal12/2(SignalData)
  BuildSignal9/1(SignalBytes) -> Mux/11
  BuildSignal10/1(SignalBytes) -> Mux/12
  BuildSignal11/1(SignalBytes) -> Mux/13
  BuildSignal12/1(SignalBytes) -> Mux/14
  BuildSignal18/1(SignalBytes) -> Mux/15
  Data Type Conversion15/1 -> BuildSignal14/1(SignalNo)
  Enumerated Constant15/1 -> Data Type Conversion15/1
  state/1 -> BuildSignal14/2(SignalData)
  powerI2R/1 -> BuildSignal15/2(SignalData)
  Enumerated Constant16/1 -> Data Type Conversion16/1
  Data Type Conversion16/1 -> BuildSignal15/1(SignalNo)
  Data Type Conversion17/1 -> BuildSignal16/1(SignalNo)
  Enumerated Constant17/1 -> Data Type Conversion17/1
  powerNet/1 -> BuildSignal16/2(SignalData)
  BuildSignal14/1(SignalBytes) -> Mux/16
  BuildSignal15/1(SignalBytes) -> Mux/17
  BuildSignal16/1(SignalBytes) -> Mux/18
  powerNetMean/1 -> BuildSignal17/2(SignalData)
  Enumerated Constant18/1 -> Data Type Conversion18/1
  Data Type Conversion18/1 -> BuildSignal17/1(SignalNo)
  BuildSignal17/1(SignalBytes) -> Mux/19
  Enumerated Constant19/1 -> Data Type Conversion19/1
  Data Type Conversion19/1 -> BuildSignal18/1(SignalNo)
  powerNetMovingAvg/1 -> BuildSignal18/2(SignalData)

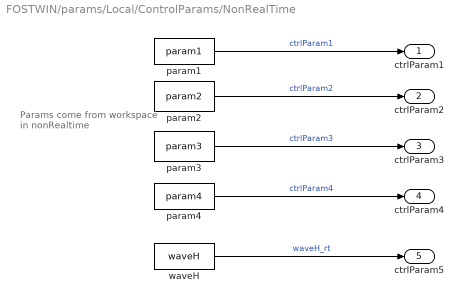
== system FOSTWIN/params/Local/ControlParams/NonRealTime ==
  note: Params come from workspace in nonRealtime
  param1 : Constant  Value=param1  OutDataTypeStr=Inherit: Inherit via back propagation  SampleTime=Ts
  param2 : Constant  Value=param2  SampleTime=Ts
  param3 : Constant  Value=param3  SampleTime=Ts
  param4 : Constant  Value=param4  VectorParams1D=off  SampleTime=Ts
  waveH : Constant  Value=waveH  SampleTime=Ts
  ctrlParam1 : Outport
  ctrlParam2 : Outport  Port=2
  ctrlParam3 : Outport  Port=3
  ctrlParam4 : Outport  Port=4
  ctrlParam5 : Outport  Port=5
  wires:
  param3/1 -> ctrlParam3/1  "ctrlParam3"
  param1/1 -> ctrlParam1/1  "ctrlParam1"
  param2/1 -> ctrlParam2/1  "ctrlParam2"
  param4/1 -> ctrlParam4/1  "ctrlParam4"
  waveH/1 -> ctrlParam5/1  "waveH_rt"

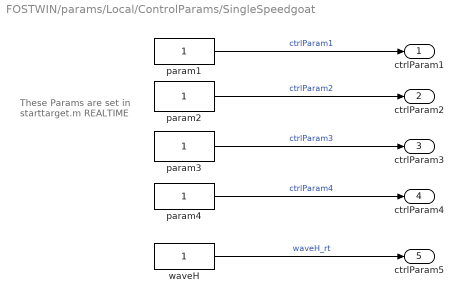
== system FOSTWIN/params/Local/ControlParams/SingleSpeedgoat ==
  note: These Params are set in starttarget.m
      | REALTIME
  param1 : Constant  OutDataTypeStr=Inherit: Inherit via back propagation  SampleTime=Ts
  param2 : Constant  SampleTime=Ts
  param3 : Constant  SampleTime=Ts
  param4 : Constant  VectorParams1D=off  SampleTime=Ts
  waveH : Constant  SampleTime=Ts
  ctrlParam1 : Outport
  ctrlParam2 : Outport  Port=2
  ctrlParam3 : Outport  Port=3
  ctrlParam4 : Outport  Port=4
  ctrlParam5 : Outport  Port=5
  wires:
  param3/1 -> ctrlParam3/1  "ctrlParam3"
  param1/1 -> ctrlParam1/1  "ctrlParam1"
  param2/1 -> ctrlParam2/1  "ctrlParam2"
  param4/1 -> ctrlParam4/1  "ctrlParam4"
  waveH/1 -> ctrlParam5/1  "waveH_rt"

== system FOSTWIN/ouput/Remote/Send UDP Data/BuildDataPckts/BuildSignal0 ==
  SignalNo : Inport
  SignalData : Inport  Port=2
  "Byte Packing " : slrealtimeutilitieslib/Byte Packing  MaskPackedDataType=uint8  MaskUnpackedDataTypes={'uint8','uint8','single'}  MaskAlignment=1
  Data Type Conversion : DataTypeConversion  OutDataTypeStr=uint8  SaturateOnIntegerOverflow=off  RndMeth=Floor
  Enumerated Constant : simulink/Sources/Enumerated Constant  OutDataTypeStr=Enum: pcktID  Value=pcktID.data  SampleTime=inf
  SignalBytes : Outport
  wires:
  SignalNo/1 -> "Byte Packing "/2
  SignalData/1 -> "Byte Packing "/3
  "Byte Packing "/1 -> SignalBytes/1
  Enumerated Constant/1 -> Data Type Conversion/1
  Data Type Conversion/1 -> "Byte Packing "/1

== system FOSTWIN/ouput/Remote/Send UDP Data/BuildDataPckts/BuildSignal1 ==
  SignalNo : Inport
  SignalData : Inport  Port=2
  "Byte Packing " : slrealtimeutilitieslib/Byte Packing  MaskPackedDataType=uint8  MaskUnpackedDataTypes={'uint8','uint8','single'}  MaskAlignment=1
  Data Type Conversion : DataTypeConversion  OutDataTypeStr=uint8  SaturateOnIntegerOverflow=off  RndMeth=Floor
  Enumerated Constant : simulink/Sources/Enumerated Constant  OutDataTypeStr=Enum: pcktID  Value=pcktID.data  SampleTime=inf
  SignalBytes : Outport
  wires:
  Data Type Conversion/1 -> "Byte Packing "/1
  Enumerated Constant/1 -> Data Type Conversion/1
  "Byte Packing "/1 -> SignalBytes/1
  SignalData/1 -> "Byte Packing "/3
  SignalNo/1 -> "Byte Packing "/2

== system FOSTWIN/ouput/Remote/Send UDP Data/BuildDataPckts/BuildSignal10 ==
  SignalNo : Inport
  SignalData : Inport  Port=2
  "Byte Packing " : slrealtimeutilitieslib/Byte Packing  MaskPackedDataType=uint8  MaskUnpackedDataTypes={'uint8','uint8','single'}  MaskAlignment=1
  Data Type Conversion : DataTypeConversion  OutDataTypeStr=uint8  SaturateOnIntegerOverflow=off  RndMeth=Floor
  Enumerated Constant : simulink/Sources/Enumerated Constant  OutDataTypeStr=Enum: pcktID  Value=pcktID.data  SampleTime=inf
  SignalBytes : Outport
  wires:
  Data Type Conversion/1 -> "Byte Packing "/1
  Enumerated Constant/1 -> Data Type Conversion/1
  "Byte Packing "/1 -> SignalBytes/1
  SignalData/1 -> "Byte Packing "/3
  SignalNo/1 -> "Byte Packing "/2

== system FOSTWIN/ouput/Remote/Send UDP Data/BuildDataPckts/BuildSignal11 ==
  SignalNo : Inport
  SignalData : Inport  Port=2
  "Byte Packing " : slrealtimeutilitieslib/Byte Packing  MaskPackedDataType=uint8  MaskUnpackedDataTypes={'uint8','uint8','single'}  MaskAlignment=1
  Data Type Conversion : DataTypeConversion  OutDataTypeStr=uint8  SaturateOnIntegerOverflow=off  RndMeth=Floor
  Enumerated Constant : simulink/Sources/Enumerated Constant  OutDataTypeStr=Enum: pcktID  Value=pcktID.data  SampleTime=inf
  SignalBytes : Outport
  wires:
  SignalNo/1 -> "Byte Packing "/2
  SignalData/1 -> "Byte Packing "/3
  "Byte Packing "/1 -> SignalBytes/1
  Enumerated Constant/1 -> Data Type Conversion/1
  Data Type Conversion/1 -> "Byte Packing "/1

== system FOSTWIN/ouput/Remote/Send UDP Data/BuildDataPckts/BuildSignal12 ==
  SignalNo : Inport
  SignalData : Inport  Port=2
  "Byte Packing " : slrealtimeutilitieslib/Byte Packing  MaskPackedDataType=uint8  MaskUnpackedDataTypes={'uint8','uint8','single'}  MaskAlignment=1
  Data Type Conversion : DataTypeConversion  OutDataTypeStr=uint8  SaturateOnIntegerOverflow=off  RndMeth=Floor
  Enumerated Constant : simulink/Sources/Enumerated Constant  OutDataTypeStr=Enum: pcktID  Value=pcktID.data  SampleTime=inf
  SignalBytes : Outport
  wires:
  Data Type Conversion/1 -> "Byte Packing "/1
  Enumerated Constant/1 -> Data Type Conversion/1
  "Byte Packing "/1 -> SignalBytes/1
  SignalData/1 -> "Byte Packing "/3
  SignalNo/1 -> "Byte Packing "/2
